simulink model "Valve_test"  (R2015b)
settings: Solver=ode23tb  StartTime=0.0  StopTime=100  RelTol=1e-3
libraries: DAEMOT_Lib x5, simulink x1
settings Model: Creator=mwillms4  LastModifiedBy=mwillms4

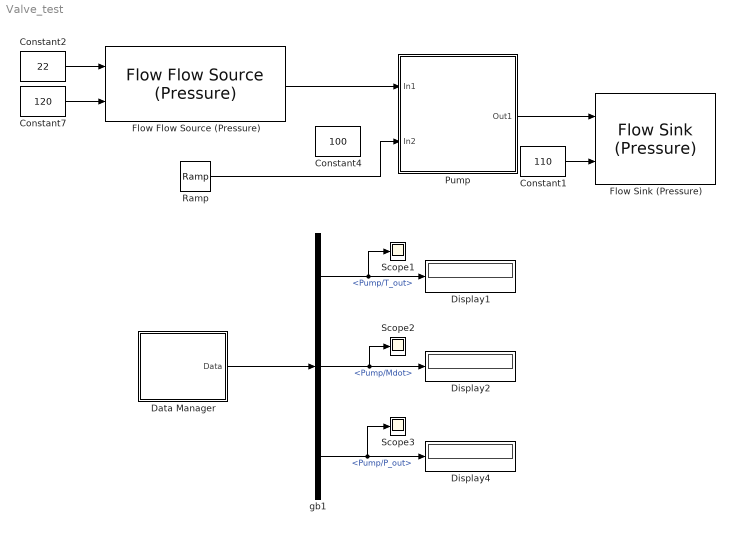
== system Valve_test ==
  Constant1 : Constant  Value=110
  Constant2 : Constant  Value=22
  Constant4 : Constant  Value=100
  Constant7 : Constant  Value=120
  Data Manager : Subsystem  AncestorBlock=DAEMOT_Lib/Support Functions/Data Manager  mask{null=0}
      mask init:
      | set_param(gcb, 'LinkStatus', 'inactive')    % disable the library link
      settings: OpenFcn=data_manager
      mask Display: str ='Pump/T_out\nPump/Mdot\nPump/P_out'; fprintf(str)
  Display1 : Display
  Display2 : Display
  Display4 : Display
  Flow Flow Source (Pressure) : DAEMOT_Lib/Components/Flow Flow Source (Pressure)  M_ext=on  M=0  T_ext=on  T=0  P_ext=on  P=0
  Flow Sink (Pressure) : DAEMOT_Lib/Components/Flow Sink (Pressure)  M_ext=on  M=0  T_ext=on  T=0  P_ext=on  P=0
  Pump : Subsystem  mask(Liquid Pump){fld=Fuel, SG=0.8, P_init=110, T_init=22, H=0, D=13*1e-3, C_v=5, k_v=1e-4, L=0.1, t=0.0015, E=2.4e6, v=5e-6}
      mask prompts: fld "Fluid Type"; SG "Fluid Specific Gravity"; P_init "Intial Outlet Pressure [kPa]"; T_init "Intial Outlet Temperature [°C]"; H "Heat Transfer Coefficient [W/m²K]"; D "Pipe Internal Diameter [m]"; C_v "Valve Coefficient, Cv [~]"; k_v "Valve Constant [~]"; L "Pipe Length [m]"; t "Tube Wall Thickness [m]"; E "Tube Modulus of Elasticity [kPa]"; v "Tube Poisson Ratio [-]"
      mask help: Tracks the time rate of change of fluid temperature, mass flow rate, and power consumption.
      mask init:
      | load('Fluids.mat');
      | Fluid = eval(['Fluid.',fld]);
      settings: OpenFcn=|
      | load('Fluids.mat');
      | Set_Fluid_Popup_Names( Fluid )
      mask TypeOptions fld: Fuel | Water | Air | PG50
      mask DialogControl Container15 Prompt: Component Sizing - Nominal Values
      mask Display:
      | %image(imread('Valve.jpg'))
      | 
      | text(0.5,0.95,['{\bf ',fld,' Valve}'],'TexMode','on','horizontalAlignment', 'center')
      | text(0.5,0.1,['{-----}'],'TexMode','on','horizontalAlignment', 'center')
      | 
      | port_label('input',1,'Flow In')
      | port_label('input',2,'Opening [%]')
      | port_label('output',1,'Flow Out')
  Ramp : simulink/Sources/Ramp  slope=1  start=0  X0=0
  Scope1 : Scope
  Scope2 : Scope
  Scope3 : Scope
  gb1 : BusSelector  OutputSignals=Pump/T_out,Pump/Mdot,Pump/P_out
  wires:
  Data Manager/1(Data) -> gb1/1
  gb1/1 -> Scope1/1, Display1/1  "<Pump/T_out>"
  gb1/2 -> Scope2/1, Display2/1  "<Pump/Mdot>"
  Flow Flow Source (Pressure)/1 -> Pump/1(In1)
  Constant7/1 -> Flow Flow Source (Pressure)/2
  Constant2/1 -> Flow Flow Source (Pressure)/1
  gb1/3 -> Scope3/1, Display4/1  "<Pump/P_out>"
  Pump/1(Out1) -> Flow Sink (Pressure)/1
  Constant1/1 -> Flow Sink (Pressure)/2
  Ramp/1 -> Pump/2(In2)

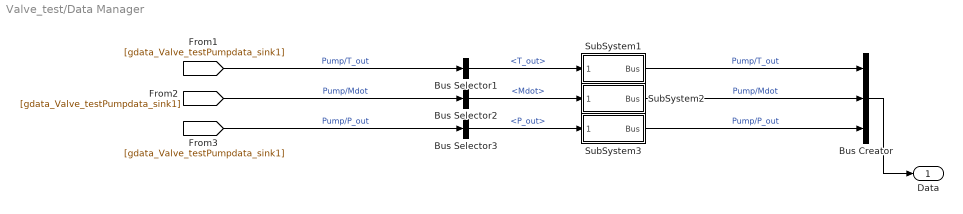
== system Valve_test/Data Manager ==
  Bus Creator : BusCreator  Inputs=3
  Bus Selector1 : BusSelector  OutputSignals=T_out
  Bus Selector2 : BusSelector  OutputSignals=Mdot
  Bus Selector3 : BusSelector  OutputSignals=P_out
  SubSystem1 : Subsystem
  SubSystem2 : Subsystem
  SubSystem3 : Subsystem
  Data : Outport
  wires:
  Bus Creator/1 -> Data/1
  [gdata_Valve_testPumpdata_sink1] -> Bus Selector1/1  "Pump/T_out"
  Bus Selector1/1 -> SubSystem1/1(Rename)  "<T_out>"
  SubSystem1/1(Bus) -> Bus Creator/1  "Pump/T_out"
  [gdata_Valve_testPumpdata_sink1] -> Bus Selector2/1  "Pump/Mdot"
  Bus Selector2/1 -> SubSystem2/1(Rename)  "<Mdot>"
  SubSystem2/1(Bus) -> Bus Creator/2  "Pump/Mdot"
  [gdata_Valve_testPumpdata_sink1] -> Bus Selector3/1  "Pump/P_out"
  Bus Selector3/1 -> SubSystem3/1(Rename)  "<P_out>"
  SubSystem3/1(Bus) -> Bus Creator/3  "Pump/P_out"

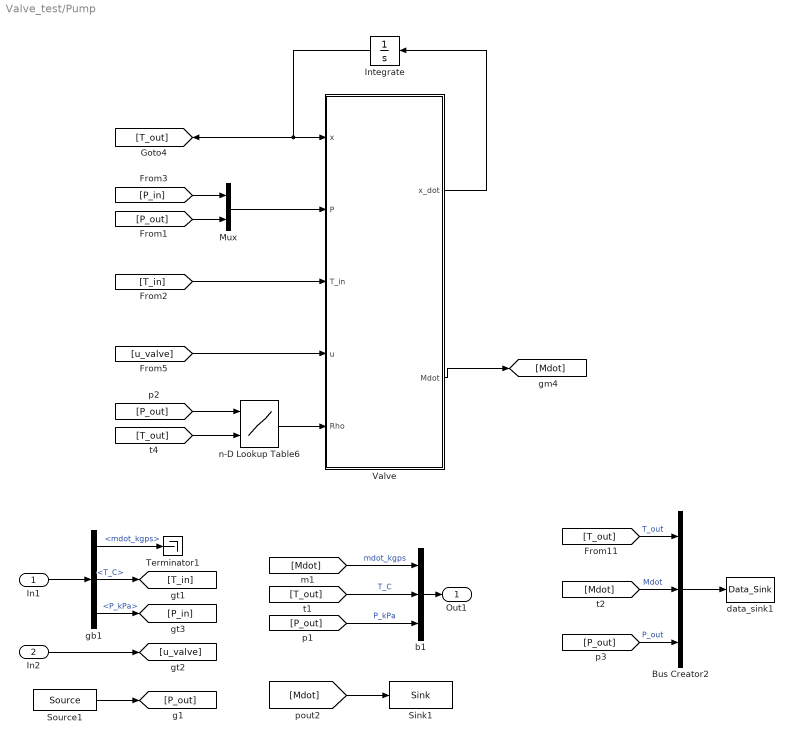
== system Valve_test/Pump ==
  In1 : Inport
  In2 : Inport  Port=2
  Bus Creator2 : BusCreator  Inputs=3
  Integrate : Integrator  InitialCondition=[T_init]
  Mux : Mux  Inputs=2
  Sink1 : DAEMOT_Lib/Support Functions/Sink
  Source1 : DAEMOT_Lib/Support Functions/Source
  Terminator1 : Terminator
  Valve : MATLAB Function  TreatAsAtomicUnit=on
  b1 : BusCreator  Inputs=3
  data_sink1 : DAEMOT_Lib/Support Functions/Data_Sink
  gb1 : BusSelector  OutputSignals=mdot_kgps,T_C,P_kPa
  n-D Lookup Table6 : Lookup_n-D  BreakpointsForDimension1=Fluid.P  BreakpointsForDimension2=Fluid.T  BreakpointsForDimension3=[5, 7]  Table=Fluid.Rho_pt  ExtrapMethod=Clip  UseLastTableValue=on  RndMeth=Simplest  InputSameDT=on
  Out1 : Outport
  wires:
  Integrate/1 -> Valve/1(x), [T_out]
  Valve/2(Mdot) -> [Mdot]
  [P_out] -> Bus Creator2/3  "P_out"
  [T_in] -> Valve/3(T_in)
  [T_out] -> n-D Lookup Table6/2
  [P_out] -> n-D Lookup Table6/1
  n-D Lookup Table6/1 -> Valve/5(Rho)
  Valve/1(x_dot) -> Integrate/1
  [P_in] -> Mux/1
  [Mdot] -> Bus Creator2/2  "Mdot"
  [T_out] -> Bus Creator2/1  "T_out"
  Bus Creator2/1 -> data_sink1/1
  [u_valve] -> Valve/4(u)
  In2/1 -> [u_valve]
  Source1/1 -> [P_out]
  [Mdot] -> Sink1/1
  gb1/3 -> [P_in]  "<P_kPa>"
  [P_out] -> b1/3  "P_kPa"
  In1/1 -> gb1/1
  gb1/1 -> Terminator1/1  "<mdot_kgps>"
  [T_out] -> b1/2  "T_C"
  gb1/2 -> [T_in]  "<T_C>"
  [Mdot] -> b1/1  "mdot_kgps"
  b1/1 -> Out1/1
  [P_out] -> Mux/2
  Mux/1 -> Valve/2(P)

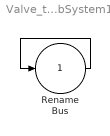
== system Valve_test/Data Manager/SubSystem1 ==
  Rename : Inport
  Bus : Outport
  wires:
  Rename/1 -> Bus/1

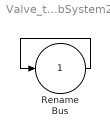
== system Valve_test/Data Manager/SubSystem2 ==
  Rename : Inport
  Bus : Outport
  wires:
  Rename/1 -> Bus/1

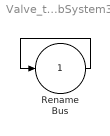
== system Valve_test/Data Manager/SubSystem3 ==
  Rename : Inport
  Bus : Outport
  wires:
  Rename/1 -> Bus/1

== matlab function Valve_test/Pump/Valve ==
  data: x input; x_dot output; Mdot output; P input; T_in input; u input; Rho input; D parameter; C_v parameter; L parameter; SG parameter; k_v parameter
function [x_dot,Mdot]= Valve(x,P,T_in,u,Rho,D,C_v,L,SG, k_v)


% Constants and Conversions
V       = L*pi*D^2/4;               % Volume
g       = 9.81;                     % Gravitational acceleration
% C_v     = 5;                        % valve flow coefficient
% SG      = 0.8;                      % specific gravity of JP8

% Parse states
T       = x(1);                     % Temperature of the tank
% P       = x(2);                     % Pressure at bottom of the tank

% Additional intermediate variable calculations
dP      = (P(1) - P(2));               % Pressure difference [kPa]
u       = u/100;                    % valve input [0-1]

Q       = k_v*u*C_v *sqrt_Lip(dP/SG);     % volumetric flow rate

% Calculate outputs
Mdot    = Rho*Q;                    % Mass flow rate [kg/s]
         
% Calculate state derivatives
T_dot   = Mdot*(T_in-T)/(V*Rho);    % Valve outlet temperature 
% P_dot   = (Mdot-Mdot_down)/(V*Rho*(1/E_fluid+D*(1-v/2)/(t*E))); % Valve outlet pressure

% Mux state derivatives
% x_dot  = [T_dot,P_dot];
x_dot  = [T_dot];
end
